simulink model "Lab_2_Exercise"  (R2018a)
settings: Solver=VariableStepAuto  StartTime=0.0  StopTime=10.0  RelTol=1e-3
settings Model: Creator=WIN  LastModifiedBy=WIN

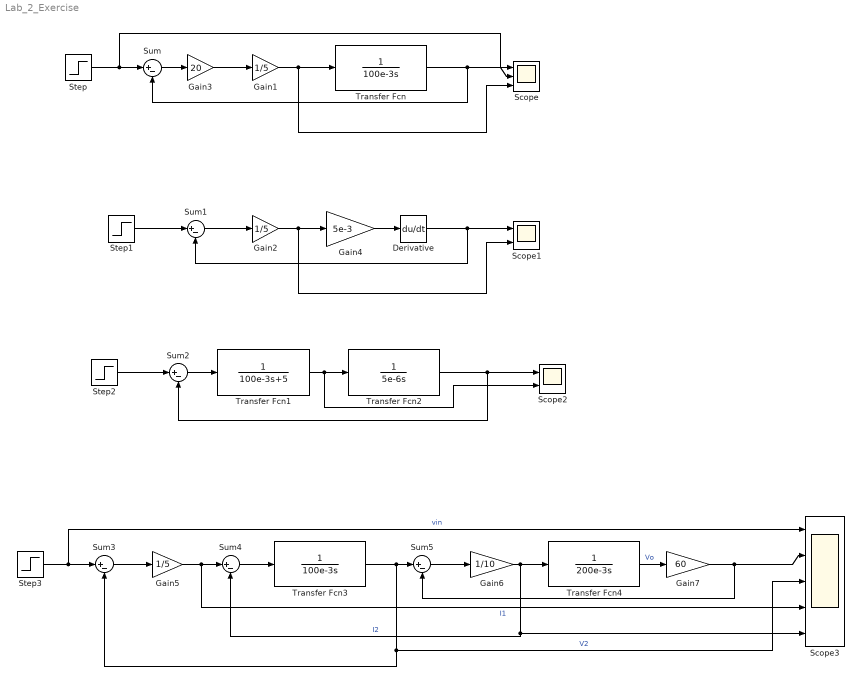
== system Lab_2_Exercise ==
  Derivative : Derivative
  Gain1 : Gain  Gain=1/5
  Gain2 : Gain  Gain=1/5
  Gain3 : Gain  Gain=20
  Gain4 : Gain  Gain=5e-3
  Gain5 : Gain  Gain=1/5
  Gain6 : Gain  Gain=1/10
  Gain7 : Gain  Gain=60
  Scope : Scope  NumInputPorts=3
  Scope1 : Scope  NumInputPorts=2
  Scope2 : Scope  NumInputPorts=2
  Scope3 : Scope  NumInputPorts=5
  Step{,1..3} (4 alike) : Step  SampleTime=0
  Sum{,1..5} (6 alike) : Sum  Inputs=|+-
  Transfer Fcn : TransferFcn  Denominator=[100e-3 0]
  Transfer Fcn1 : TransferFcn  Denominator=[100e-3 5]
  Transfer Fcn2 : TransferFcn  Denominator=[5e-6 0]
  Transfer Fcn3 : TransferFcn  Denominator=[100e-3 0]
  Transfer Fcn4 : TransferFcn  Denominator=[200e-3 0]
  wires:
  Sum/1 -> Gain3/1
  Step/1 -> Scope/1, Sum/1
  Gain1/1 -> Scope/3, Transfer Fcn/1
  Transfer Fcn/1 -> Scope/2, Sum/2
  Derivative/1 -> Scope1/1, Sum1/2
  Gain2/1 -> Scope1/2, Gain4/1
  Step1/1 -> Sum1/1
  Sum1/1 -> Gain2/1
  Gain3/1 -> Gain1/1
  Gain4/1 -> Derivative/1
  Step2/1 -> Sum2/1
  Sum2/1 -> Transfer Fcn1/1
  Transfer Fcn1/1 -> Scope2/2, Transfer Fcn2/1
  Transfer Fcn2/1 -> Scope2/1, Sum2/2
  Step3/1 -> Scope3/1, Sum3/1  "vin"
  Sum3/1 -> Gain5/1
  Gain5/1 -> Scope3/4, Sum4/1  "I1"
  Sum4/1 -> Transfer Fcn3/1
  Transfer Fcn3/1 -> Scope3/3, Sum3/2, Sum5/1  "V2"
  Sum5/1 -> Gain6/1
  Gain6/1 -> Scope3/5, Sum4/2, Transfer Fcn4/1  "I2"
  Transfer Fcn4/1 -> Gain7/1  "Vo"
  Gain7/1 -> Scope3/2, Sum5/2
